simulink model "untitled"  (R2020b)
settings: Solver=VariableStepAuto  StartTime=0.0  StopTime=100  MaxStep=1e-3  RelTol=1e-3
settings Model: Creator=yuqiang  LastModifiedBy=yuqiang

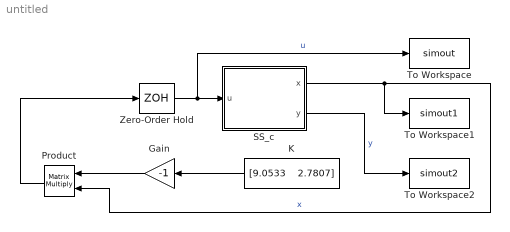
== system untitled ==
  Gain : Gain  Gain=-1
  K : Constant  Value="[9.0533    2.7807]"  VectorParams1D=off
  Product : Product  Multiplication=Matrix(*)
  SS_c : Subsystem
  To Workspace : ToWorkspace  VariableName=simout  SaveFormat=Timeseries  SampleTime=-1
  To Workspace1 : ToWorkspace  VariableName=simout1  SaveFormat=Timeseries  SampleTime=-1
  To Workspace2 : ToWorkspace  VariableName=simout2  SaveFormat=Timeseries  SampleTime=-1
  Zero-Order Hold : ZeroOrderHold  SampleTime=0.2
  wires:
  Zero-Order Hold/1 -> To Workspace/1, SS_c/1(u)  "u"
  Product/1 -> Zero-Order Hold/1
  SS_c/1(x) -> To Workspace1/1, Product/2  "x"
  K/1 -> Gain/1
  Gain/1 -> Product/1
  SS_c/2(y) -> To Workspace2/1  "y"

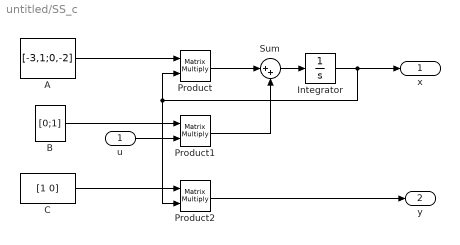
== system untitled/SS_c ==
  u : Inport
  A : Constant  Value=[-3,1;0,-2]  VectorParams1D=off
  B : Constant  Value=[0;1]  VectorParams1D=off
  C : Constant  Value=[1 0]  VectorParams1D=off
  Integrator : Integrator  InitialCondition=[1;0]
  Product : Product  Multiplication=Matrix(*)
  Product1 : Product  Multiplication=Matrix(*)
  Product2 : Product  Multiplication=Matrix(*)
  Sum : Sum  Inputs=|++
  x : Outport
  y : Outport  Port=2
  wires:
  u/1 -> Product1/2
  Sum/1 -> Integrator/1
  Product2/1 -> y/1
  Product/1 -> Sum/1
  A/1 -> Product/1
  B/1 -> Product1/1
  C/1 -> Product2/1
  Product1/1 -> Sum/2
  Integrator/1 -> x/1, Product/2, Product2/2
